simulink model "PEMFuelCellSystem"  (R2025b)
settings: Solver=VariableStepAuto  StartTime=0.0  StopTime=2500  RelTol=1e-3  AbsTol=1e-3
model workspace: external: MATLAB File PEMFuelCellSystemParameters.m (data not in the file)
values from neighbouring files (symbols this model uses):
  anode_tube_D = 0.01    [PEMFuelCellSystemParameters.m]
  cathode_tube_D = 0.05    [PEMFuelCellSystemParameters.m]
  comp_rpm_TLU = [0, 1800, 3600]    [PEMFuelCellSystemParameters.m]
  coolant_num_layers = 20    [PEMFuelCellSystemParameters.m]
  coolant_num_passes = 12    [PEMFuelCellSystemParameters.m]
  coolant_tube_D = 0.05    [PEMFuelCellSystemParameters.m]
  coolant_w_channels = 1    [PEMFuelCellSystemParameters.m]
  env_p = 0.101325    [PEMFuelCellSystemParameters.m]
  env_T = 20    [PEMFuelCellSystemParameters.m]
  N2_T = [-56.55, -50:10:-10, -5:1:5, 10:10:350]    [PEMFuelCellSystemParameters.m]
  radiator_air_area_fins = 2 * radiator_N_fins * radiator_W * radiator_gap_H    (= 11.5625)    [PEMFuelCellSystemParameters.m]
  radiator_air_area_primary = 2 * (radiator_N_tubes - 1) * radiator_W * (radiator_L + radiator_gap_H)    (= 1.223125)    [PEMFuelCellSystemParameters.m]
  radiator_eta_fin = 0.7    [PEMFuelCellSystemParameters.m]
  radiator_N_tubes = 25    [PEMFuelCellSystemParameters.m]
  radiator_rho = 2700    [PEMFuelCellSystemParameters.m]
  radiator_t_wall = 1e-4    (= 0.0001)    [PEMFuelCellSystemParameters.m]
  radiator_tube_H = 0.0015    [PEMFuelCellSystemParameters.m]
  radiator_W = 0.025    [PEMFuelCellSystemParameters.m]
  stack_area = 280    [PEMFuelCellSystemParameters.m]
  stack_iL = 1.4    [PEMFuelCellSystemParameters.m]
  stack_mea_rho = 1800    [PEMFuelCellSystemParameters.m]
  stack_num_cells = 400    [PEMFuelCellSystemParameters.m]
  stack_num_channels = 8    [PEMFuelCellSystemParameters.m]
  stack_t_gdl = 250    [PEMFuelCellSystemParameters.m]
  stack_t_membrane = 125    [PEMFuelCellSystemParameters.m]
  stack_w_channels = 1    [PEMFuelCellSystemParameters.m]
libraries: fl_lib x83, nesl_utility x23, slpidlib x2, simulink x1
(part 1 of 3)
CloseFcn:
  | try,close(h1_PEMFuelCellSystem),end
  | clear h1_PEMFuelCellSystem
  | try,close(h2_PEMFuelCellSystem),end
  | clear h2_PEMFuelCellSystem
  | try,close(h3_PEMFuelCellSystem),end
  | clear h3_PEMFuelCellSystem
  | try,close(h4_PEMFuelCellSystem),end
  | clear h4_PEMFuelCellSystem
  | try,close(h5_PEMFuelCellSystem),end
  | clear h5_PEMFuelCellSystem
  | 
  | clear tout simlog_PEMFuelCellSystem
Description:
  | PEM Fuel Cell System
settings Model: Creator=The MathWorks, Inc.  LastModifiedBy=The MathWorks, Inc.
settings SolverCC: AutoScaleAbsTol=off  MaxConsecutiveMinStep=2  AlgebraicLoopSolver=TrustRegion  MaxZcPerStep=1.0
settings DataIOCC: ReturnWorkspaceOutputs=off
settings DebuggingCC: UnconnectedInputMsg=warning  UnconnectedOutputMsg=warning  UnconnectedLineMsg=warning  SymbolicDimsDataTypeCodeGenerationDiagnostic=none
settings ModelReferenceCC: EnableRefExpFcnMdlSchedulingChecks=on
settings SFSimCC: CustomCodeUndefinedFunction=UseInterfaceOnly
settings RTWCC: GPUComputeCapability=3.5  DLArmComputeVersion=19.05
settings SimscapeCC: SimscapeLogType=all  SimscapeLogSimulationStatistics=on  SimscapeLogName=simlog_PEMFuelCellSystem  SimscapeLogDataHistory=20000.0

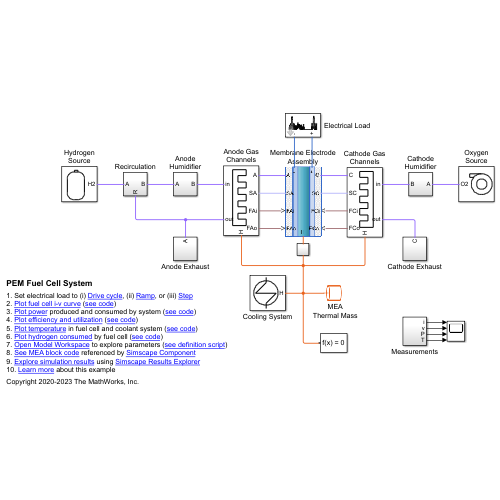
[thumbnail: Simulink's stored preview of the top-level diagram]
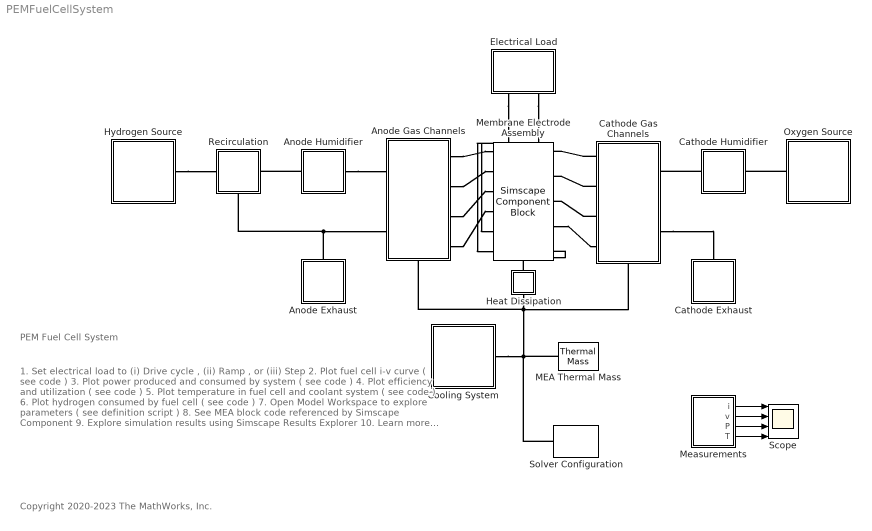
== system PEMFuelCellSystem ==
  note: PEM Fuel Cell System
  note: 1. Set electrical load to (i) Drive cycle , (ii) Ramp , or (iii) Step
      | 2. Plot fuel cell i-v curve ( see code )
      | 3. Plot power produced and consumed by system ( see code )
      | 4. Plot efficiency and utilization ( see code )
      | 5. Plot temperature in fuel cell and coolant system ( see code )
      | 6. Plot hydrogen consumed by fuel cell ( see code )
      | 7. Open Model Workspace to explore parameters ( see definition script )
      | 8. See MEA block code referenced by Simscape Component
      | 9. Explore simulation results using Simscape Results Explorer
      | 10. Learn more about this example
  note: Copyright 2020-2023 The MathWorks, Inc.
  Anode Humidifier : Subsystem  Tag=PublishSubsystem
  Anode Exhaust : Subsystem  Tag=PublishSubsystem
      settings: PortSchema="{\"entries\":[{\"content\":{\"sides\":[{\"content\":{\"connectorIds\":[]},\"type\":\"ConnectorPlacement.EquallySpacedRectSide\",\"uuid\":\"6344d1cf-22ea-4a51-9588-07afca0fac15\"},{\"content\":{\"connectorIds\":[],\"side\":\"RIGHT\"},\"type\":\"ConnectorPlacement.EquallySpacedRectSide\",\"uuid\":\"a3908f81-9410-4056-87cd-9faba76d3fb8\"},{\"content\":{\"connectorIds\":[\"LConn1\"],\"side\":\"TOP\"},\"type\":\"ConnectorPlacement.EquallySpacedRectSide\",\"uuid\":\"a1c9e24d-adb9-4361-8e9b-feafccbbdb81\"}]},\"type\":\"ConnectorPlacement.EquallySpacedConnector\",\"uuid\":\"d5180d8f-18a0-491d-9fff-909db43c9aea\"}],\"packageUris\":[\"http://schema.mathworks.com/mf0/Connector/R2020b\"],\"version\":\"1.0\"}"
  Anode Gas Channels : Subsystem  Tag=PublishSubsystem
      settings: PortSchema="{\"entries\":[{\"content\":{\"sides\":[{\"content\":{\"connectorIds\":[\"LConn1\",\"LConn2\"]},\"type\":\"ConnectorPlacement.EquallySpacedRectSide\",\"uuid\":\"f0c92738-2de1-40ac-9e4a-670524600aa2\"},{\"content\":{\"connectorIds\":[\"RConn1\",\"RConn2\",\"RConn3\",\"RConn4\"],\"side\":\"RIGHT\"},\"type\":\"ConnectorPlacement.EquallySpacedRectSide\",\"uuid\":\"f0ed995d-2dce-4bd6-9faa-b1cb502a30b1\"},{\"content\":{\"connectorIds\":[],\"side\":\"TOP\"},\"type\":\"ConnectorPlacement.EquallySpacedRectSide\",\"uuid\":\"b5d2d698-46b6-42b5-a767-bb9f1790aa28\"},{\"content\":{\"connectorIds\":[\"RConn5\"],\"side\":\"BOTTOM\"},\"type\":\"ConnectorPlacement.EquallySpacedRectSide\",\"uuid\":\"3e8c99a3-0044-43a9-bacb-b652445e4ac6\"}]},\"type\":\"ConnectorPlacement.EquallySpacedConnector\",\"uuid\":\"912925fb-ca80-4fe6-8a1d-a2308cfd6f88\"}],\"packageUris\":[\"http://schema.mathworks.com/mf0/Connector/R2020b\"],\"version\":\"1.0\"}"
      mask Display:
      | plot(0, 0)
      | plot(100, 100)
      | 
      | x1 = 25;
      | x2 = 65;
      | y1 = 23;
      | y2 = 95;
      | xt = 15;
      | yt = 9;
      | 
      | x_pattern = [x2 x2    x1+xt x1+xt   x1+xt   x2     ];
      | y_pattern = [y2 y2-yt y2-yt y2-2*yt y2-2*yt y2-2*yt];
      | 
      | plot([x1 x1 x2 x_pattern x_pattern      x_pattern      x_pattern         x2    x1], ...
      |      [y1-yt y2 y2 y_pattern y_pattern-2*yt y_pattern-4*yt y_pattern-6*yt y1-yt y1-yt])
  Cathode Humidifier : Subsystem  Tag=PublishSubsystem
  Cathode Exhaust : Subsystem  Tag=PublishSubsystem
      settings: PortSchema="{\"entries\":[{\"content\":{\"sides\":[{\"content\":{\"connectorIds\":[]},\"type\":\"ConnectorPlacement.EquallySpacedRectSide\",\"uuid\":\"6344d1cf-22ea-4a51-9588-07afca0fac15\"},{\"content\":{\"connectorIds\":[],\"side\":\"RIGHT\"},\"type\":\"ConnectorPlacement.EquallySpacedRectSide\",\"uuid\":\"a3908f81-9410-4056-87cd-9faba76d3fb8\"},{\"content\":{\"connectorIds\":[\"LConn1\"],\"side\":\"TOP\"},\"type\":\"ConnectorPlacement.EquallySpacedRectSide\",\"uuid\":\"a1c9e24d-adb9-4361-8e9b-feafccbbdb81\"}]},\"type\":\"ConnectorPlacement.EquallySpacedConnector\",\"uuid\":\"d5180d8f-18a0-491d-9fff-909db43c9aea\"}],\"packageUris\":[\"http://schema.mathworks.com/mf0/Connector/R2020b\"],\"version\":\"1.0\"}"
  Cathode Gas Channels : Subsystem  Tag=PublishSubsystem
      settings: PortSchema="{\"entries\":[{\"content\":{\"sides\":[{\"content\":{\"connectorIds\":[\"LConn1\",\"LConn2\",\"LConn3\",\"LConn4\"]},\"type\":\"ConnectorPlacement.EquallySpacedRectSide\",\"uuid\":\"d09155df-6760-40de-80f3-d532399b6b43\"},{\"content\":{\"connectorIds\":[\"RConn1\",\"RConn2\"],\"side\":\"RIGHT\"},\"type\":\"ConnectorPlacement.EquallySpacedRectSide\",\"uuid\":\"8f76bd4e-30c2-4c8b-860a-78c10353bd22\"},{\"content\":{\"connectorIds\":[],\"side\":\"TOP\"},\"type\":\"ConnectorPlacement.EquallySpacedRectSide\",\"uuid\":\"7de91a32-4f26-479e-bbec-b6009a288b8f\"},{\"content\":{\"connectorIds\":[\"RConn3\"],\"side\":\"BOTTOM\"},\"type\":\"ConnectorPlacement.EquallySpacedRectSide\",\"uuid\":\"b696b46e-4734-4c8a-bae1-7c8793078c6b\"}]},\"type\":\"ConnectorPlacement.EquallySpacedConnector\",\"uuid\":\"30d7c265-b676-4649-8112-8a94c6c095da\"}],\"packageUris\":[\"http://schema.mathworks.com/mf0/Connector/R2020b\"],\"version\":\"1.0\"}"
      mask Display:
      | plot(0, 0)
      | plot(100, 100)
      | 
      | x1 = 35;
      | x2 = 75;
      | y1 = 23;
      | y2 = 95;
      | xt = 15;
      | yt = 9;
      | 
      | x_pattern = [x1 x1    x2-xt x2-xt   x2-xt   x1     ];
      | y_pattern = [y2 y2-yt y2-yt y2-2*yt y2-2*yt y2-2*yt];
      | 
      | plot([x2 x2 x1 x_pattern x_pattern      x_pattern      x_pattern         x1    x2], ...
      |      [y1-yt y2 y2 y_pattern y_pattern-2*yt y_pattern-4*yt y_pattern-6*yt y1-yt y1-yt])
  Cooling System : Subsystem  Tag=PublishSubsystem
      mask Display:
      | plot(0, 0)
      | plot(100, 100)
      | 
      | n = 80;
      | r = 35;
      | 
      | x = 45;
      | y = 50;
      | t = 5;
      | 
      | plot(cos(linspace(0, 2*pi, n))*r + x, sin(linspace(0, 2*pi, n))*r + y)
      | 
      | plot([x x x-r+t x+r-t x x], [y+r+2*t y+r-t y y y-r+t y-r-2*t])
  Electrical Load : Subsystem  Tag=PublishSubsystem  mask(Electrical Load){input_type=Drive cycle}
      mask prompts: input_type "Select one of the following scenarios:"
      settings: PortSchema="{\"entries\":[{\"content\":{\"sides\":[{\"content\":{\"connectorIds\":[]},\"type\":\"ConnectorPlacement.EquallySpacedRectSide\",\"uuid\":\"cf26c57a-4aaa-4eca-a1cf-dab3379228b7\"},{\"content\":{\"connectorIds\":[],\"side\":\"RIGHT\"},\"type\":\"ConnectorPlacement.EquallySpacedRectSide\",\"uuid\":\"bd4a28c6-f8d3-4492-9f61-a12eb17ccdd3\"},{\"content\":{\"connectorIds\":[],\"side\":\"TOP\"},\"type\":\"ConnectorPlacement.EquallySpacedRectSide\",\"uuid\":\"7f54a4db-ccf4-4e3a-a135-4ada067d241f\"},{\"content\":{\"connectorIds\":[\"RConn1\",\"RConn2\"],\"side\":\"BOTTOM\"},\"type\":\"ConnectorPlacement.EquallySpacedRectSide\",\"uuid\":\"8817983d-3f79-43b3-9594-6d12f7dcf066\"}]},\"type\":\"ConnectorPlacement.EquallySpacedConnector\",\"uuid\":\"79253ea6-cd7f-4983-840a-f5cee3a4dd91\"}],\"packageUris\":[\"http://schema.mathworks.com/mf0/Connector/R2020b\"],\"version\":\"1.0\"}"
      mask TypeOptions input_type: Drive cycle | Ramp | Step
      mask Callback input_type:
      | activeVariant = get_param(gcb, 'input_type');
      | set_param([gcb '/Inputs'], 'OverrideUsingVariant', activeVariant)
      mask Display:
      | blk = get_param([gcb, '/Inputs'], 'CompiledActiveChoiceBlock');
      | eval(get_param(blk, 'MaskDisplay'))
  Heat Dissipation : Subsystem
      settings: PortSchema="{\"entries\":[{\"content\":{\"sides\":[{\"content\":{\"connectorIds\":[]},\"type\":\"ConnectorPlacement.EquallySpacedRectSide\",\"uuid\":\"40b2385a-b20e-464f-8016-3228e4acac4a\"},{\"content\":{\"connectorIds\":[],\"side\":\"RIGHT\"},\"type\":\"ConnectorPlacement.EquallySpacedRectSide\",\"uuid\":\"0e95dc4b-d2da-4ab6-a6e9-e2cb275776ce\"},{\"content\":{\"connectorIds\":[\"LConn1\"],\"side\":\"TOP\"},\"type\":\"ConnectorPlacement.EquallySpacedRectSide\",\"uuid\":\"0f5995c7-26f6-433d-889b-dea78bcd2b2a\"},{\"content\":{\"connectorIds\":[\"RConn1\"],\"side\":\"BOTTOM\"},\"type\":\"ConnectorPlacement.EquallySpacedRectSide\",\"uuid\":\"a2ee1c19-f9e9-4dbd-a9ff-92feea387e85\"}]},\"type\":\"ConnectorPlacement.EquallySpacedConnector\",\"uuid\":\"721753ea-9ada-4c74-8c6f-50b905d96904\"}],\"packageUris\":[\"http://schema.mathworks.com/mf0/Connector/R2020b\"],\"version\":\"1.0\"}"
  Hydrogen Source : Subsystem  Tag=PublishSubsystem
      mask Display:
      | plot(0, 0)
      | plot(100, 100)
      | 
      | n = 20;
      | r = 20;
      | x1 = 15;
      | x2 = 65;
      | y1 = 5;
      | y2 = 85;
      | 
      | plot([x1 x1], [y1+r y2-r])
      | plot([x1+r x2-r], [y2 y2])
      | plot([x2 x2], [y2-r y1+r])
      | plot([x2-r x1+r], [y1 y1])
      | 
      | plot(cos(linspace(pi/2, pi, n))*r + x1+r, sin(linspace(pi/2, pi, n))*r + y2-r)
      | plot(cos(linspace(0, pi/2, n))*r + x2-r, sin(linspace(0, pi/2, n))*r + y2-r)
      | plot(cos(linspace(3*pi/2, 2*pi, n))*r + x2-r, sin(linspace(3*pi/2, 2*pi, n))*r + y1+r)
      | plot(cos(linspace(pi, 3*pi/2, n))*r + x1+r, sin(linspace(pi, 3*pi/2, n))*r + y1+r)
      | 
      | plot([-5 -5 5 5] + (x1+x2)/2, [0 5 5 0] + y2)
  MEA Thermal Mass : fl_lib/Thermal/Thermal Elements/Thermal Mass  mass_type=foundation.enum.constant_variable.constant  mass=stack_mea_rho * stack_area*1e-4 * (stack_t_membrane + 2*stack_t_gdl)*1e-6 * stack_num_cells kg  sp_heat=stack_mea_cp J/kg/K  mass_min=1e-6 kg  num_ports=foundation.enum.numPorts2.one  m_specify=off  m_priority=High  m=1 kg  m_nominal_specify=off  m_nominal_value=1  m_nominal_unit=kg  T_specify=on  T_priority=High  T=env_T degC  T_nominal_specify=off  T_nominal_value=1  T_nominal_unit=K  Q_specify=off  Q_priority=None  Q=0 W  Q_nominal_specify=off  Q_nominal_value=1  Q_nominal_unit=W
  Measurements : Subsystem
  Membrane Electrode Assembly : SimscapeComponentBlock  SourceFile=FuelCell  ComponentPath=FuelCell  ComponentVariants="[\"FuelCell\"]"  ComponentVariantNames="[\"FuelCell\"]"  ClassName=FuelCell  SchemaVersion=1  N_cell=stack_num_cells  area_cell=stack_area cm^2  t_membrane=stack_t_membrane um  t_gdl_A=stack_t_gdl um  t_gdl_C=stack_t_gdl um  io=stack_io A/cm^2  iL=stack_iL A/cm^2  alpha=stack_alpha  D_H2O_gdl_A=stack_D_gdl cm^2/s  D_H2O_gdl_C=stack_D_gdl cm^2/s  rho_membrane=stack_membrane_rho kg/m^3  M_membrane=stack_membrane_MW kg/mol  i_specify=off  i_priority=None  i=0 A  i_nominal_specify=off  i_nominal_value=1  i_nominal_unit=A  Q_specify=off  Q_priority=None  Q=0 W  Q_nominal_specify=off  Q_nominal_value=1  Q_nominal_unit=W  a_H2O_acl_specify=off  a_H2O_acl_priority=None  a_H2O_acl=0.5  a_H2O_acl_nominal_specify=off  a_H2O_acl_nominal_value=1  a_H2O_acl_nominal_unit=1  a_H2O_ccl_specify=off  a_H2O_ccl_priority=None  a_H2O_ccl=0.5  a_H2O_ccl_nominal_specify=off  a_H2O_ccl_nominal_value=1  a_H2O_ccl_nominal_unit=1
      settings: CopyFcn=simscape.sscblock.internal.componentBlockCallback(gcbh,'COPY')  PreCopyFcn=simscape.sscblock.internal.componentBlockCallback(gcbh,'PRECOPY')  PreDeleteFcn=simscape.sscblock.internal.componentBlockCallback(gcbh,'PREDELETE')  InternalSimscapePortConfiguration="{\"Bottom\":[{\"id\":\"H\",\"label\":\"H\",\"type\":\"foundation.thermal.thermal\"}],\"Left\":[{\"id\":\"A\",\"label\":\"A\",\"type\":\"foundation.moist_air.moist_air\"},{\"id\":\"SA\",\"label\":\"SA\",\"type\":\"foundation.moist_air.moist_air_source\"},{\"id\":\"FAi\",\"label\":\"FAi\",\"type\":\"input\"},{\"id\":\"FAo\",\"label\":\"FAo\",\"type\":\"input\"}],\"Right\":[{\"id\":\"C\",\"label\":\"C\",\"type\":\"foundation.moist_air.moist_air\"},{\"id\":\"SC\",\"label\":\"SC\",\"type\":\"foundation.moist_air.moist_air_source\"},{\"id\":\"FCi\",\"label\":\"FCi\",\"type\":\"input\"},{\"id\":\"FCo\",\"label\":\"FCo\",\"type\":\"input\"}],\"Top\":[{\"id\":\"n\",\"label\":\"-\",\"type\":\"foundation.electrical.electrical\"},{\"id\":\"p\",\"label\":\"+\",\"type\":\"foundation.electrical.electrical\"}]}"
      mask Type: Fuel Cell
  Oxygen Source : Subsystem  Tag=PublishSubsystem
      mask Display:
      | plot(0, 0)
      | plot(100, 100)
      | 
      | n = 80;
      | r1 = 15;
      | r2 = 30;
      | 
      | plot(cos(linspace(0, 2*pi, n))*r1 + 65, sin(linspace(0, 2*pi, n))*r1 + 50)
      | plot(cos(linspace(0, 2*pi, n))*r2 + 65, sin(linspace(0, 2*pi, n))*r2 + 50)
      | 
      | plot([65 30 30 42], [80 80 70 70])
  Recirculation : Subsystem  Tag=PublishSubsystem
      settings: PortSchema="{\"entries\":[{\"content\":{\"sides\":[{\"content\":{\"connectorIds\":[\"LConn1\"]},\"type\":\"ConnectorPlacement.EquallySpacedRectSide\",\"uuid\":\"a905d28b-4136-4e4b-b56f-ff4ef454860e\"},{\"content\":{\"connectorIds\":[\"RConn1\"],\"side\":\"RIGHT\"},\"type\":\"ConnectorPlacement.EquallySpacedRectSide\",\"uuid\":\"7d453241-460d-4f71-8108-f868ae96b726\"},{\"content\":{\"connectorIds\":[],\"side\":\"TOP\"},\"type\":\"ConnectorPlacement.EquallySpacedRectSide\",\"uuid\":\"5de5a8e7-eaa9-43ea-9e3e-e109b24be5c4\"},{\"content\":{\"connectorIds\":[\"RConn2\"],\"side\":\"BOTTOM\"},\"type\":\"ConnectorPlacement.EquallySpacedRectSide\",\"uuid\":\"9c44ad98-d3d2-40d8-a226-ad16e20687d9\"}]},\"type\":\"ConnectorPlacement.EquallySpacedConnector\",\"uuid\":\"be431bc9-ad83-41b5-a4a3-7fe11e97fedb\"}],\"packageUris\":[\"http://schema.mathworks.com/mf0/Connector/R2020b\"],\"version\":\"1.0\"}"
  Scope : Scope  NumInputPorts=4
      settings: Title=Current (A)  ActiveDisplayYMinimum=-34.06707  ActiveDisplayYMaximum=306.60365
  Solver Configuration : nesl_utility/Solver Configuration  PhysicalDomain=network_engine_domain  SubClassName=solver  LeftPortType=input  RightPortType=generic  Tones=[]  Harmonics=[]  SimulateNoise=off  Profile=off  UseLocalSampling=off  EnableSwitchedLinearOptims=on  FrequencyDomain=off  UseCCode=off  RelTol=0.001  AbsTol=1e-06  MinStep=1e-09  ToWorkspace=off  RevertToSquareIcSolve=off  NumHomotopyIterations=100  PhasorMode=off  PhasorModeNumHarmonics=1  ConsistencySolver=NEWTON_XTOL_AFTER_FTOL  IndexReductionMethod=DerivativeReplacement  DoDC=off  ResidualTolerance=1e-09  ConsistencyTolSource=GLOBAL  ConsistencyAbsTol=0.001  ConsistencyRelTol=0.001  ConsistencyTolFactor=0.001  UseLocalSolver=off  LocalSolverChoice=NE_BACKWARD_EULER_ADVANCER  ResolveIndetEquations=on  FunctionEvalNumThread=1  LocalSolverSampleTime=0.001  DoFixedCost=off  MaxNonlinIter=3  MaxModeIter=2  ComputeImpulses=off  ImpulseIterations=2  LinearAlgebra=auto  LinearAlgebraNumThread=0  EquationFormulation=NE_TIME_EF  DelaysMemoryBudget=1024  AutomaticFiltering=on  FilteringTimeConstant=0.001  PartitionStorageMethod=AS_NEEDED  PartitionMemoryBudget=1024  PartitionMethod=ROBUST  MultibodyUseLocalSolver=off  MultibodyLocalSolverChoice=ODE1  MultibodyLocalSolverSampleTime=0.001
  wires:
  Measurements/1(i) -> Scope/1
  Measurements/2(v) -> Scope/2
  Measurements/3(P) -> Scope/3
  Measurements/4(T) -> Scope/4
  connections:
  Cathode Gas Channels/RConn2 -- Cathode Exhaust/LConn1
  Cathode Humidifier/LConn1 -- Cathode Gas Channels/RConn1
  Anode Gas Channels/RConn1 -- Membrane Electrode Assembly/LConn1
  Anode Gas Channels/RConn2 -- Membrane Electrode Assembly/LConn2
  Anode Gas Channels/RConn3 -- Membrane Electrode Assembly/LConn3
  Cathode Gas Channels/LConn1 -- Membrane Electrode Assembly/RConn1
  Cathode Gas Channels/LConn2 -- Membrane Electrode Assembly/RConn2
  Cathode Gas Channels/LConn3 -- Membrane Electrode Assembly/RConn3
  Anode Exhaust/LConn1 -- Recirculation/RConn2 -- Anode Gas Channels/LConn2
  Oxygen Source/LConn1 -- Cathode Humidifier/RConn1
  Electrical Load/RConn1 -- Membrane Electrode Assembly/LConn5
  Electrical Load/RConn2 -- Membrane Electrode Assembly/LConn6
  Anode Gas Channels/RConn4 -- Membrane Electrode Assembly/LConn4
  Membrane Electrode Assembly/RConn4 -- Cathode Gas Channels/LConn4
  Anode Humidifier/RConn1 -- Anode Gas Channels/LConn1
  Hydrogen Source/RConn1 -- Recirculation/LConn1
  Anode Humidifier/LConn1 -- Recirculation/RConn1
  MEA Thermal Mass/LConn1 -- Solver Configuration/RConn1 -- Heat Dissipation/RConn1 -- Anode Gas Channels/RConn5 -- Cathode Gas Channels/RConn3 -- Cooling System/RConn1
  Heat Dissipation/LConn1 -- Membrane Electrode Assembly/RConn5

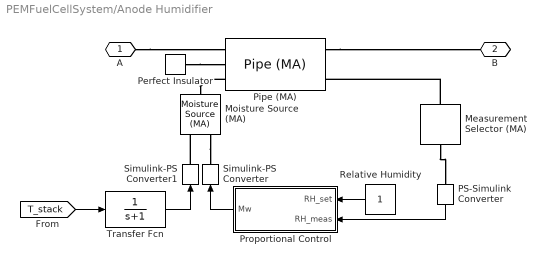
== system PEMFuelCellSystem/Anode Humidifier ==
  Measurement Selector (MA) : fl_lib/Moist Air/Sensors/Measurement Selector (MA)  moisture_spec=foundation.enum.moisture_spec.relative_humidity  trace_gas_spec=foundation.enum.trace_gas_spec.mole_fraction
      settings: InternalSimscapePortConfiguration="{\"Bottom\":[],\"Left\":[{\"id\":\"F\",\"label\":\"F\",\"type\":\"input\"}],\"Right\":[{\"id\":\"P\",\"label\":\"P\",\"type\":\"output\"},{\"id\":\"T\",\"label\":\"T\",\"type\":\"output\"},{\"id\":\"W\",\"label\":\"W\",\"type\":\"output\"},{\"id\":\"G\",\"label\":\"G\",\"type\":\"output\"},{\"id\":\"D\",\"label\":\"D\",\"type\":\"output\"}],\"Top\":[]}"
  Moisture Source (MA) : fl_lib/Moist Air/Sources/Moisture & Trace Gas Sources/Moisture Source (MA)  source_type=foundation.enum.constant_controlled.controlled  moisture_source_spec=foundation.enum.MoistureSourceSpec.WaterVapor  vapor_from_liquid=false  moisture_mass_flow=0 kg/s  temperature_spec=foundation.enum.temperature_spec.atmospheric  moisture_temperature=293.15 K  Phi_S_specify=off  Phi_S_priority=None  Phi_S=0 kW  Phi_S_nominal_specify=off  Phi_S_nominal_value=1  Phi_S_nominal_unit=kW  mdot_w_S_specify=off  mdot_w_S_priority=None  mdot_w_S=0 kg/s  mdot_w_S_nominal_specify=off  mdot_w_S_nominal_value=1  mdot_w_S_nominal_unit=kg/s  mdot_d_S_specify=off  mdot_d_S_priority=None  mdot_d_S=0 kg/s  mdot_d_S_nominal_specify=off  mdot_d_S_nominal_value=1  mdot_d_S_nominal_unit=kg/s
      settings: InternalSimscapePortConfiguration="{\"Bottom\":[],\"Left\":[{\"id\":\"S\",\"label\":\"S\",\"type\":\"foundation.moist_air.moist_air_source\"}],\"Right\":[{\"id\":\"M\",\"label\":\"M\",\"type\":\"input\"},{\"id\":\"T\",\"label\":\"T\",\"type\":\"input\"}],\"Top\":[]}"
  PS-Simulink Converter : nesl_utility/PS-Simulink Converter  PhysicalDomain=network_engine_domain  SubClassName=ps_output  LeftPortType=input  RightPortType=output  PseudoPeriodic=off  Frequencies=[]  VectorFormat=1-D array  Unit=1  AffineConversion=off
  Perfect Insulator : fl_lib/Thermal/Thermal Elements/Perfect Insulator  T_specify=off  T_priority=None  T=0 K  T_nominal_specify=off  T_nominal_value=1  T_nominal_unit=K
  Pipe (MA) : fl_lib/Moist Air/Elements/Pipe (MA)  length=0.25 m  area=pi*0.05^2/4 m^2  Dh=0.05 m  length_add=0.1 m  roughness=15e-6 m  Re_lam=2000  Re_tur=4000  shape_factor=64  Nu_lam=3.66  wall_condensation=simscape.enum.onoff.off  RH_ws=1  time_constant_cond=1e-3 s  time_constant_evap=1e-3 s  fraction_entrained=1  moisture_trace_gas_source=foundation.enum.moisture_trace_gas_source.controlled  moisture_source_spec=foundation.enum.MoistureSourceSpec.WaterVapor  vapor_from_liquid=false  moisture_mass_flow=0 kg/s  moisture_temperature_spec=foundation.enum.temperature_spec.atmospheric  moisture_temperature=293.15 K  trace_gas_mass_flow=0 kg/s  trace_gas_temperature_spec=foundation.enum.temperature_spec.atmospheric  trace_gas_temperature=293.15 K  p_init=env_p MPa  p_init_priority=foundation.enum.Priority.High  T_init=env_T degC  T_init_priority=foundation.enum.Priority.High  humidity_spec=foundation.enum.HumiditySpec.RelativeHumidity  RH_init=0  RH_init_priority=foundation.enum.Priority.High  x_w_init=0  x_w_init_priority=foundation.enum.Priority.None  y_w_init=0  y_w_init_priority=foundation.enum.Priority.None  HR_init=0  HR_init_priority=foundation.enum.Priority.None  Tw_init=287 K  Tw_init_priority=foundation.enum.Priority.High  trace_gas_spec=foundation.enum.trace_gas_spec.mole_fraction  x_g_init=0  x_g_init_priority=foundation.enum.Priority.None  y_g_init=tank_yH2  y_g_init_priority=foundation.enum.Priority.High  r_d_init=0  r_d_init_priority=foundation.enum.Priority.High
      settings: InternalSimscapePortConfiguration="{\"Bottom\":[],\"Left\":[{\"id\":\"A\",\"label\":\"A\",\"type\":\"foundation.moist_air.moist_air\"},{\"id\":\"H\",\"label\":\"H\",\"type\":\"foundation.thermal.thermal\"},{\"id\":\"S\",\"label\":\"S\",\"type\":\"foundation.moist_air.moist_air_source\"}],\"Right\":[{\"id\":\"B\",\"label\":\"B\",\"type\":\"foundation.moist_air.moist_air\"},{\"id\":\"W\",\"label\":\"W\",\"type\":\"output\"},{\"id\":\"F\",\"label\":\"F\",\"type\":\"output\"}],\"Top\":[]}"
  Proportional Control : Subsystem
  Relative Humidity : Constant
  Simulink-PS Converter : nesl_utility/Simulink-PS Converter  PhysicalDomain=network_engine_domain  SubClassName=ps_input  LeftPortType=input  RightPortType=output  PseudoPeriodic=off  Frequencies=[]  NoiseDistribution=none  NoiseParameters=[]  Unit=kg/s  AffineConversion=off  FilteringAndDerivatives=provide  SimscapeFilterOrder=1  InputFilterTimeConstant=0.001  UdotUserProvided=0
  Simulink-PS Converter1 : nesl_utility/Simulink-PS Converter  PhysicalDomain=network_engine_domain  SubClassName=ps_input  LeftPortType=input  RightPortType=output  PseudoPeriodic=off  Frequencies=[]  NoiseDistribution=none  NoiseParameters=[]  Unit=degC  AffineConversion=on  FilteringAndDerivatives=provide  SimscapeFilterOrder=1  InputFilterTimeConstant=0.001  UdotUserProvided=0
  Transfer Fcn : TransferFcn  Denominator=[1 1]
  A : PMIOPort  Side=Left
  B : PMIOPort  Port=2  Side=Right
  wires:
  Transfer Fcn/1 -> Simulink-PS Converter1/1
  [T_stack] -> Transfer Fcn/1
  Relative Humidity/1 -> Proportional Control/1(RH_set)
  PS-Simulink Converter/1 -> Proportional Control/2(RH_meas)
  Proportional Control/1(Mw) -> Simulink-PS Converter/1
  connections:
  Moisture Source (MA)/RConn1 -- Simulink-PS Converter/RConn1
  Measurement Selector (MA)/LConn1 -- Pipe (MA)/RConn3
  Simulink-PS Converter1/RConn1 -- Moisture Source (MA)/RConn2
  Pipe (MA)/LConn3 -- Moisture Source (MA)/LConn1
  Perfect Insulator/LConn1 -- Pipe (MA)/LConn2
  Pipe (MA)/RConn1 -- B/RConn1
  A/RConn1 -- Pipe (MA)/LConn1
  Measurement Selector (MA)/RConn3 -- PS-Simulink Converter/LConn1

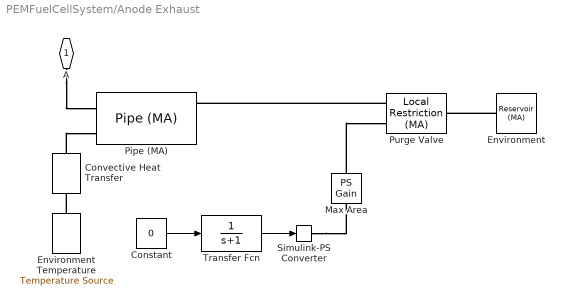
== system PEMFuelCellSystem/Anode Exhaust ==
  Constant : Constant  Value=0
  Convective Heat Transfer : fl_lib/Thermal/Thermal Elements/Convective Heat Transfer  thermal_type=foundation.enum.constant_variable.constant  area=pi*anode_tube_D*1 m^2  heat_tr_coeff=20 W/(m^2 * K)  min_heat_tr_coeff=1e-3 W/(K*m^2)  T_specify=off  T_priority=None  T=0 K  T_nominal_specify=off  T_nominal_value=1  T_nominal_unit=K  Q_specify=off  Q_priority=None  Q=0 W  Q_nominal_specify=off  Q_nominal_value=1  Q_nominal_unit=W
  Environment : fl_lib/Moist Air/Elements/Reservoir (MA)  pressure_input=false  pressure_spec=foundation.enum.pressure_spec.specified  reservoir_pressure=env_p MPa  temperature_input=false  temperature_spec=foundation.enum.temperature_spec.specified  reservoir_temperature=env_T degC  humidity_input=false  humidity_spec=foundation.enum.HumiditySpec.RelativeHumidity  reservoir_RH=0  reservoir_x_w=0.01  reservoir_y_w=0.01  reservoir_HR=0.01  reservoir_Tw=287 K  trace_gas_input=false  trace_gas_spec=foundation.enum.trace_gas_spec.mole_fraction  reservoir_x_g=0.001  reservoir_y_g=tank_yH2  water_droplets_input=false  reservoir_r_d=0  RH_ws=1  area_A=pi*anode_tube_D^2/4 m^2  input_error_spec=foundation.enum.input_range_error.warn
  Environment Temperature : fl_lib/Thermal/Thermal Sources/Temperature Source  temperature=env_T degC
  Max Area : fl_lib/Physical Signals/Functions/PS Gain  gain=pi*(0.2*anode_tube_D)^2/4 m^2
  Pipe (MA) : fl_lib/Moist Air/Elements/Pipe (MA)  length=1 m  area=pi*anode_tube_D^2/4 m^2  Dh=anode_tube_D m  length_add=0.1 m  roughness=15e-6 m  Re_lam=2000  Re_tur=4000  shape_factor=64  Nu_lam=3.66  wall_condensation=simscape.enum.onoff.off  RH_ws=1  time_constant_cond=1e-3 s  time_constant_evap=1e-3 s  fraction_entrained=1  moisture_trace_gas_source=foundation.enum.moisture_trace_gas_source.none  moisture_source_spec=foundation.enum.MoistureSourceSpec.WaterVapor  vapor_from_liquid=false  moisture_mass_flow=0 kg/s  moisture_temperature_spec=foundation.enum.temperature_spec.atmospheric  moisture_temperature=293.15 K  trace_gas_mass_flow=0 kg/s  trace_gas_temperature_spec=foundation.enum.temperature_spec.atmospheric  trace_gas_temperature=293.15 K  p_init=env_p MPa  p_init_priority=foundation.enum.Priority.High  T_init=env_T degC  T_init_priority=foundation.enum.Priority.High  humidity_spec=foundation.enum.HumiditySpec.RelativeHumidity  RH_init=0  RH_init_priority=foundation.enum.Priority.High  x_w_init=0  x_w_init_priority=foundation.enum.Priority.None  y_w_init=0  y_w_init_priority=foundation.enum.Priority.None  HR_init=0  HR_init_priority=foundation.enum.Priority.None  Tw_init=287 K  Tw_init_priority=foundation.enum.Priority.High  trace_gas_spec=foundation.enum.trace_gas_spec.mole_fraction  x_g_init=0  x_g_init_priority=foundation.enum.Priority.None  y_g_init=tank_yH2  y_g_init_priority=foundation.enum.Priority.High  r_d_init=0  r_d_init_priority=foundation.enum.Priority.High
  Purge Valve : fl_lib/Moist Air/Elements/Local Restriction (MA)  restriction_type=foundation.enum.restriction_type.variable  restriction_area=0.001 m^2  min_area=pi*(1e-4*anode_tube_D)^2/4 m^2  max_area=pi*(0.2*anode_tube_D)^2/4 m^2  area=pi*anode_tube_D^2/4 m^2  Cd=0.64  B_lam=0.999
  Simulink-PS Converter : nesl_utility/Simulink-PS Converter  PhysicalDomain=network_engine_domain  SubClassName=ps_input  LeftPortType=input  RightPortType=output  PseudoPeriodic=off  Frequencies=[]  NoiseDistribution=none  NoiseParameters=[]  Unit=1  AffineConversion=off  FilteringAndDerivatives=provide  SimscapeFilterOrder=1  InputFilterTimeConstant=0.001  UdotUserProvided=0
  Transfer Fcn : TransferFcn  Denominator=[1 1]
  A : PMIOPort  Side=Left
  wires:
  Constant/1 -> Transfer Fcn/1
  Transfer Fcn/1 -> Simulink-PS Converter/1
  connections:
  Environment/LConn1 -- Purge Valve/RConn1
  A/RConn1 -- Pipe (MA)/LConn1
  Purge Valve/LConn1 -- Pipe (MA)/RConn1
  Simulink-PS Converter/RConn1 -- Max Area/LConn1
  Max Area/RConn1 -- Purge Valve/LConn2
  Convective Heat Transfer/LConn1 -- Pipe (MA)/LConn2
  Environment Temperature/LConn1 -- Convective Heat Transfer/RConn1

== system PEMFuelCellSystem/Anode Gas Channels ==
  note: connection to share anode fluid properties only
  Pipe (MA) : fl_lib/Moist Air/Elements/Pipe (MA)  length=sqrt(stack_area) / 2 cm  area=stack_w_channels^2 * stack_num_channels * stack_num_cells cm^2  Dh=stack_w_channels cm  length_add=1 cm  roughness=15e-6 m  Re_lam=2000  Re_tur=4000  shape_factor=64  Nu_lam=3.66  wall_condensation=simscape.enum.onoff.off  RH_ws=1  time_constant_cond=1e-3 s  time_constant_evap=1e-3 s  fraction_entrained=1  moisture_trace_gas_source=foundation.enum.moisture_trace_gas_source.none  moisture_source_spec=foundation.enum.MoistureSourceSpec.WaterVapor  vapor_from_liquid=false  moisture_mass_flow=0 kg/s  moisture_temperature_spec=foundation.enum.temperature_spec.atmospheric  moisture_temperature=293.15 K  trace_gas_mass_flow=0 kg/s  trace_gas_temperature_spec=foundation.enum.temperature_spec.atmospheric  trace_gas_temperature=293.15 K  p_init=env_p MPa  p_init_priority=foundation.enum.Priority.High  T_init=env_T degC  T_init_priority=foundation.enum.Priority.High  humidity_spec=foundation.enum.HumiditySpec.RelativeHumidity  RH_init=0  RH_init_priority=foundation.enum.Priority.High  x_w_init=0  x_w_init_priority=foundation.enum.Priority.None  y_w_init=0  y_w_init_priority=foundation.enum.Priority.None  HR_init=0  HR_init_priority=foundation.enum.Priority.None  Tw_init=287 K  Tw_init_priority=foundation.enum.Priority.High  trace_gas_spec=foundation.enum.trace_gas_spec.mole_fraction  x_g_init=0  x_g_init_priority=foundation.enum.Priority.None  y_g_init=tank_yH2  y_g_init_priority=foundation.enum.Priority.High  r_d_init=0  r_d_init_priority=foundation.enum.Priority.High
  Pipe (MA)1 : fl_lib/Moist Air/Elements/Pipe (MA)  length=sqrt(stack_area) / 2 cm  area=stack_w_channels^2 * stack_num_channels * stack_num_cells cm^2  Dh=stack_w_channels cm  length_add=1 cm  roughness=15e-6 m  Re_lam=2000  Re_tur=4000  shape_factor=64  Nu_lam=3.66  wall_condensation=simscape.enum.onoff.off  RH_ws=1  time_constant_cond=1e-3 s  time_constant_evap=1e-3 s  fraction_entrained=1  moisture_trace_gas_source=foundation.enum.moisture_trace_gas_source.controlled  moisture_source_spec=foundation.enum.MoistureSourceSpec.WaterVapor  vapor_from_liquid=false  moisture_mass_flow=0 kg/s  moisture_temperature_spec=foundation.enum.temperature_spec.atmospheric  moisture_temperature=293.15 K  trace_gas_mass_flow=0 kg/s  trace_gas_temperature_spec=foundation.enum.temperature_spec.atmospheric  trace_gas_temperature=293.15 K  p_init=env_p MPa  p_init_priority=foundation.enum.Priority.High  T_init=env_T degC  T_init_priority=foundation.enum.Priority.High  humidity_spec=foundation.enum.HumiditySpec.RelativeHumidity  RH_init=0  RH_init_priority=foundation.enum.Priority.High  x_w_init=0  x_w_init_priority=foundation.enum.Priority.None  y_w_init=0  y_w_init_priority=foundation.enum.Priority.None  HR_init=0  HR_init_priority=foundation.enum.Priority.None  Tw_init=287 K  Tw_init_priority=foundation.enum.Priority.High  trace_gas_spec=foundation.enum.trace_gas_spec.mole_fraction  x_g_init=0  x_g_init_priority=foundation.enum.Priority.None  y_g_init=tank_yH2  y_g_init_priority=foundation.enum.Priority.High  r_d_init=0  r_d_init_priority=foundation.enum.Priority.High
      settings: InternalSimscapePortConfiguration="{\"Bottom\":[],\"Left\":[{\"id\":\"A\",\"label\":\"A\",\"type\":\"foundation.moist_air.moist_air\"},{\"id\":\"H\",\"label\":\"H\",\"type\":\"foundation.thermal.thermal\"},{\"id\":\"S\",\"label\":\"S\",\"type\":\"foundation.moist_air.moist_air_source\"}],\"Right\":[{\"id\":\"B\",\"label\":\"B\",\"type\":\"foundation.moist_air.moist_air\"},{\"id\":\"W\",\"label\":\"W\",\"type\":\"output\"},{\"id\":\"F\",\"label\":\"F\",\"type\":\"output\"}],\"Top\":[]}"
  in : PMIOPort  Side=Left
  out : PMIOPort  Port=2  Side=Left
  A : PMIOPort  Port=3  Side=Right
  SA : PMIOPort  Port=4  Side=Right
  FAi : PMIOPort  Port=5  Side=Right
  FAo : PMIOPort  Port=6  Side=Right
  H : PMIOPort  Port=7  Side=Right
  connections:
  Pipe (MA)/LConn1 -- in/RConn1
  Pipe (MA)1/RConn1 -- out/RConn1
  Pipe (MA)/LConn2 -- Pipe (MA)1/LConn2 -- H/RConn1
  FAo/RConn1 -- Pipe (MA)1/RConn3
  Pipe (MA)/RConn3 -- FAi/RConn1
  Pipe (MA)1/LConn3 -- SA/RConn1
  Pipe (MA)/RConn1 -- Pipe (MA)1/LConn1 -- A/RConn1

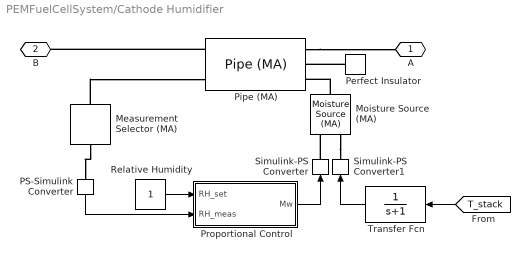
== system PEMFuelCellSystem/Cathode Humidifier ==
  Measurement Selector (MA) : fl_lib/Moist Air/Sensors/Measurement Selector (MA)  moisture_spec=foundation.enum.moisture_spec.relative_humidity  trace_gas_spec=foundation.enum.trace_gas_spec.mole_fraction
      settings: InternalSimscapePortConfiguration="{\"Bottom\":[],\"Left\":[{\"id\":\"F\",\"label\":\"F\",\"type\":\"input\"}],\"Right\":[{\"id\":\"P\",\"label\":\"P\",\"type\":\"output\"},{\"id\":\"T\",\"label\":\"T\",\"type\":\"output\"},{\"id\":\"W\",\"label\":\"W\",\"type\":\"output\"},{\"id\":\"G\",\"label\":\"G\",\"type\":\"output\"},{\"id\":\"D\",\"label\":\"D\",\"type\":\"output\"}],\"Top\":[]}"
  Moisture Source (MA) : fl_lib/Moist Air/Sources/Moisture & Trace Gas Sources/Moisture Source (MA)  source_type=foundation.enum.constant_controlled.controlled  moisture_source_spec=foundation.enum.MoistureSourceSpec.WaterVapor  vapor_from_liquid=false  moisture_mass_flow=0 kg/s  temperature_spec=foundation.enum.temperature_spec.atmospheric  moisture_temperature=293.15 K  Phi_S_specify=off  Phi_S_priority=None  Phi_S=0 kW  Phi_S_nominal_specify=off  Phi_S_nominal_value=1  Phi_S_nominal_unit=kW  mdot_w_S_specify=off  mdot_w_S_priority=None  mdot_w_S=0 kg/s  mdot_w_S_nominal_specify=off  mdot_w_S_nominal_value=1  mdot_w_S_nominal_unit=kg/s  mdot_d_S_specify=off  mdot_d_S_priority=None  mdot_d_S=0 kg/s  mdot_d_S_nominal_specify=off  mdot_d_S_nominal_value=1  mdot_d_S_nominal_unit=kg/s
      settings: InternalSimscapePortConfiguration="{\"Bottom\":[],\"Left\":[{\"id\":\"S\",\"label\":\"S\",\"type\":\"foundation.moist_air.moist_air_source\"}],\"Right\":[{\"id\":\"M\",\"label\":\"M\",\"type\":\"input\"},{\"id\":\"T\",\"label\":\"T\",\"type\":\"input\"}],\"Top\":[]}"
  PS-Simulink Converter : nesl_utility/PS-Simulink Converter  PhysicalDomain=network_engine_domain  SubClassName=ps_output  LeftPortType=input  RightPortType=output  PseudoPeriodic=off  Frequencies=[]  VectorFormat=1-D array  Unit=1  AffineConversion=off
  Perfect Insulator : fl_lib/Thermal/Thermal Elements/Perfect Insulator  T_specify=off  T_priority=None  T=0 K  T_nominal_specify=off  T_nominal_value=1  T_nominal_unit=K
  Pipe (MA) : fl_lib/Moist Air/Elements/Pipe (MA)  length=0.25 m  area=pi*0.05^2/4 m^2  Dh=0.05 m  length_add=0.1 m  roughness=15e-6 m  Re_lam=2000  Re_tur=4000  shape_factor=64  Nu_lam=3.66  wall_condensation=simscape.enum.onoff.off  RH_ws=1  time_constant_cond=1e-3 s  time_constant_evap=1e-3 s  fraction_entrained=1  moisture_trace_gas_source=foundation.enum.moisture_trace_gas_source.controlled  moisture_source_spec=foundation.enum.MoistureSourceSpec.WaterVapor  vapor_from_liquid=false  moisture_mass_flow=0 kg/s  moisture_temperature_spec=foundation.enum.temperature_spec.atmospheric  moisture_temperature=293.15 K  trace_gas_mass_flow=0 kg/s  trace_gas_temperature_spec=foundation.enum.temperature_spec.atmospheric  trace_gas_temperature=293.15 K  p_init=env_p MPa  p_init_priority=foundation.enum.Priority.High  T_init=env_T degC  T_init_priority=foundation.enum.Priority.High  humidity_spec=foundation.enum.HumiditySpec.RelativeHumidity  RH_init=env_RH  RH_init_priority=foundation.enum.Priority.High  x_w_init=0  x_w_init_priority=foundation.enum.Priority.None  y_w_init=0  y_w_init_priority=foundation.enum.Priority.None  HR_init=0  HR_init_priority=foundation.enum.Priority.None  Tw_init=287 K  Tw_init_priority=foundation.enum.Priority.High  trace_gas_spec=foundation.enum.trace_gas_spec.mole_fraction  x_g_init=0  x_g_init_priority=foundation.enum.Priority.None  y_g_init=env_yO2  y_g_init_priority=foundation.enum.Priority.High  r_d_init=0  r_d_init_priority=foundation.enum.Priority.High
      settings: InternalSimscapePortConfiguration="{\"Bottom\":[],\"Left\":[{\"id\":\"A\",\"label\":\"A\",\"type\":\"foundation.moist_air.moist_air\"},{\"id\":\"H\",\"label\":\"H\",\"type\":\"foundation.thermal.thermal\"},{\"id\":\"S\",\"label\":\"S\",\"type\":\"foundation.moist_air.moist_air_source\"}],\"Right\":[{\"id\":\"B\",\"label\":\"B\",\"type\":\"foundation.moist_air.moist_air\"},{\"id\":\"W\",\"label\":\"W\",\"type\":\"output\"},{\"id\":\"F\",\"label\":\"F\",\"type\":\"output\"}],\"Top\":[]}"
  Proportional Control : Subsystem
  Relative Humidity : Constant
  Simulink-PS Converter : nesl_utility/Simulink-PS Converter  PhysicalDomain=network_engine_domain  SubClassName=ps_input  LeftPortType=input  RightPortType=output  PseudoPeriodic=off  Frequencies=[]  NoiseDistribution=none  NoiseParameters=[]  Unit=kg/s  AffineConversion=off  FilteringAndDerivatives=provide  SimscapeFilterOrder=1  InputFilterTimeConstant=0.001  UdotUserProvided=0
  Simulink-PS Converter1 : nesl_utility/Simulink-PS Converter  PhysicalDomain=network_engine_domain  SubClassName=ps_input  LeftPortType=input  RightPortType=output  PseudoPeriodic=off  Frequencies=[]  NoiseDistribution=none  NoiseParameters=[]  Unit=degC  AffineConversion=on  FilteringAndDerivatives=provide  SimscapeFilterOrder=1  InputFilterTimeConstant=0.001  UdotUserProvided=0
  Transfer Fcn : TransferFcn  Denominator=[1 1]
  A : PMIOPort  Side=Right
  B : PMIOPort  Port=2  Side=Left
  wires:
  Transfer Fcn/1 -> Simulink-PS Converter1/1
  [T_stack] -> Transfer Fcn/1
  Proportional Control/1(Mw) -> Simulink-PS Converter/1
  Relative Humidity/1 -> Proportional Control/1(RH_set)
  PS-Simulink Converter/1 -> Proportional Control/2(RH_meas)
  connections:
  Moisture Source (MA)/RConn2 -- Simulink-PS Converter1/RConn1
  Measurement Selector (MA)/LConn1 -- Pipe (MA)/RConn3
  Simulink-PS Converter/RConn1 -- Moisture Source (MA)/RConn1
  Perfect Insulator/LConn1 -- Pipe (MA)/LConn2
  Measurement Selector (MA)/RConn3 -- PS-Simulink Converter/LConn1
  Moisture Source (MA)/LConn1 -- Pipe (MA)/LConn3
  Pipe (MA)/RConn1 -- B/RConn1
  Pipe (MA)/LConn1 -- A/RConn1

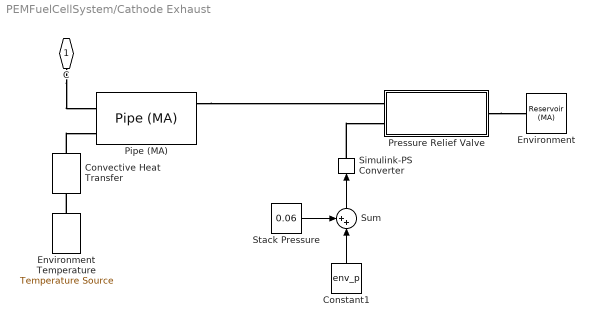
== system PEMFuelCellSystem/Cathode Exhaust ==
  Constant1 : Constant  Value=env_p
  Convective Heat Transfer : fl_lib/Thermal/Thermal Elements/Convective Heat Transfer  thermal_type=foundation.enum.constant_variable.constant  area=pi*cathode_tube_D*1 m^2  heat_tr_coeff=20 W/(m^2 * K)  min_heat_tr_coeff=1e-3 W/(K*m^2)  T_specify=off  T_priority=None  T=0 K  T_nominal_specify=off  T_nominal_value=1  T_nominal_unit=K  Q_specify=off  Q_priority=None  Q=0 W  Q_nominal_specify=off  Q_nominal_value=1  Q_nominal_unit=W
  Environment : fl_lib/Moist Air/Elements/Reservoir (MA)  pressure_input=false  pressure_spec=foundation.enum.pressure_spec.specified  reservoir_pressure=env_p MPa  temperature_input=false  temperature_spec=foundation.enum.temperature_spec.specified  reservoir_temperature=env_T degC  humidity_input=false  humidity_spec=foundation.enum.HumiditySpec.RelativeHumidity  reservoir_RH=env_RH  reservoir_x_w=0.01  reservoir_y_w=0.01  reservoir_HR=0.01  reservoir_Tw=287 K  trace_gas_input=false  trace_gas_spec=foundation.enum.trace_gas_spec.mole_fraction  reservoir_x_g=0.001  reservoir_y_g=env_yO2  water_droplets_input=false  reservoir_r_d=0  RH_ws=1  area_A=pi*cathode_tube_D^2/4 m^2  input_error_spec=foundation.enum.input_range_error.warn
  Environment Temperature : fl_lib/Thermal/Thermal Sources/Temperature Source  temperature=env_T degC
  Pipe (MA) : fl_lib/Moist Air/Elements/Pipe (MA)  length=1 m  area=pi*cathode_tube_D^2/4 m^2  Dh=cathode_tube_D m  length_add=0.1 m  roughness=15e-6 m  Re_lam=2000  Re_tur=4000  shape_factor=64  Nu_lam=3.66  wall_condensation=simscape.enum.onoff.off  RH_ws=1  time_constant_cond=1e-3 s  time_constant_evap=1e-3 s  fraction_entrained=1  moisture_trace_gas_source=foundation.enum.moisture_trace_gas_source.none  moisture_source_spec=foundation.enum.MoistureSourceSpec.WaterVapor  vapor_from_liquid=false  moisture_mass_flow=0 kg/s  moisture_temperature_spec=foundation.enum.temperature_spec.atmospheric  moisture_temperature=293.15 K  trace_gas_mass_flow=0 kg/s  trace_gas_temperature_spec=foundation.enum.temperature_spec.atmospheric  trace_gas_temperature=293.15 K  p_init=env_p MPa  p_init_priority=foundation.enum.Priority.High  T_init=env_T degC  T_init_priority=foundation.enum.Priority.High  humidity_spec=foundation.enum.HumiditySpec.RelativeHumidity  RH_init=env_RH  RH_init_priority=foundation.enum.Priority.High  x_w_init=0  x_w_init_priority=foundation.enum.Priority.None  y_w_init=0  y_w_init_priority=foundation.enum.Priority.None  HR_init=0  HR_init_priority=foundation.enum.Priority.None  Tw_init=287 K  Tw_init_priority=foundation.enum.Priority.High  trace_gas_spec=foundation.enum.trace_gas_spec.mole_fraction  x_g_init=0  x_g_init_priority=foundation.enum.Priority.None  y_g_init=env_yO2  y_g_init_priority=foundation.enum.Priority.High  r_d_init=0  r_d_init_priority=foundation.enum.Priority.High
  Pressure Relief Valve : Subsystem  Tag=PublishSubsystem  mask(Pressure Relief Valve){D=cathode_tube_D, r_min=1e-4, r_max=0.8, p_range=0.005}
      mask prompts: D "Connecting tube diameter (m)"; r_min "Min diameter ratio"; r_max "Max diameter ratio"; p_range "Pressure regulation range (MPa)"
      mask help: This subsystem models a pressure relief valve that maintains a set pressure at port A. The valve is normally closed. When the pressure is above the set pressure, it begins to open.
  Simulink-PS Converter : nesl_utility/Simulink-PS Converter  PhysicalDomain=network_engine_domain  SubClassName=ps_input  LeftPortType=input  RightPortType=output  PseudoPeriodic=off  Frequencies=[]  NoiseDistribution=none  NoiseParameters=[]  Unit=MPa  AffineConversion=off  FilteringAndDerivatives=provide  SimscapeFilterOrder=1  InputFilterTimeConstant=0.001  UdotUserProvided=0
  Stack Pressure : Constant  Value=0.06
  Sum : Sum  Inputs=++|
  C : PMIOPort  Side=Left
  wires:
  Stack Pressure/1 -> Sum/1
  Sum/1 -> Simulink-PS Converter/1
  Constant1/1 -> Sum/2
  connections:
  Pipe (MA)/RConn1 -- Pressure Relief Valve/LConn1
  C/RConn1 -- Pipe (MA)/LConn1
  Convective Heat Transfer/LConn1 -- Pipe (MA)/LConn2
  Environment Temperature/LConn1 -- Convective Heat Transfer/RConn1
  Pressure Relief Valve/RConn1 -- Environment/LConn1
  Simulink-PS Converter/RConn1 -- Pressure Relief Valve/LConn2

== system PEMFuelCellSystem/Cathode Gas Channels ==
  note: connection to share cathode fluid properties only
  Pipe (MA) : fl_lib/Moist Air/Elements/Pipe (MA)  length=sqrt(stack_area) / 2 cm  area=stack_w_channels^2 * stack_num_channels * stack_num_cells cm^2  Dh=stack_w_channels cm  length_add=1 cm  roughness=15e-6 m  Re_lam=2000  Re_tur=4000  shape_factor=64  Nu_lam=3.66  wall_condensation=simscape.enum.onoff.off  RH_ws=1  time_constant_cond=1e-3 s  time_constant_evap=1e-3 s  fraction_entrained=1  moisture_trace_gas_source=foundation.enum.moisture_trace_gas_source.none  moisture_source_spec=foundation.enum.MoistureSourceSpec.WaterVapor  vapor_from_liquid=false  moisture_mass_flow=0 kg/s  moisture_temperature_spec=foundation.enum.temperature_spec.atmospheric  moisture_temperature=293.15 K  trace_gas_mass_flow=0 kg/s  trace_gas_temperature_spec=foundation.enum.temperature_spec.atmospheric  trace_gas_temperature=293.15 K  p_init=env_p MPa  p_init_priority=foundation.enum.Priority.High  T_init=env_T degC  T_init_priority=foundation.enum.Priority.High  humidity_spec=foundation.enum.HumiditySpec.RelativeHumidity  RH_init=env_RH  RH_init_priority=foundation.enum.Priority.High  x_w_init=0  x_w_init_priority=foundation.enum.Priority.None  y_w_init=0  y_w_init_priority=foundation.enum.Priority.None  HR_init=0  HR_init_priority=foundation.enum.Priority.None  Tw_init=287 K  Tw_init_priority=foundation.enum.Priority.High  trace_gas_spec=foundation.enum.trace_gas_spec.mole_fraction  x_g_init=0  x_g_init_priority=foundation.enum.Priority.None  y_g_init=env_yO2  y_g_init_priority=foundation.enum.Priority.High  r_d_init=0  r_d_init_priority=foundation.enum.Priority.High
  Pipe (MA)1 : fl_lib/Moist Air/Elements/Pipe (MA)  length=sqrt(stack_area) / 2 cm  area=stack_w_channels^2 * stack_num_channels * stack_num_cells cm^2  Dh=stack_w_channels cm  length_add=1 cm  roughness=15e-6 m  Re_lam=2000  Re_tur=4000  shape_factor=64  Nu_lam=3.66  wall_condensation=simscape.enum.onoff.off  RH_ws=1  time_constant_cond=1e-3 s  time_constant_evap=1e-3 s  fraction_entrained=1  moisture_trace_gas_source=foundation.enum.moisture_trace_gas_source.controlled  moisture_source_spec=foundation.enum.MoistureSourceSpec.WaterVapor  vapor_from_liquid=false  moisture_mass_flow=0 kg/s  moisture_temperature_spec=foundation.enum.temperature_spec.atmospheric  moisture_temperature=293.15 K  trace_gas_mass_flow=0 kg/s  trace_gas_temperature_spec=foundation.enum.temperature_spec.atmospheric  trace_gas_temperature=293.15 K  p_init=env_p MPa  p_init_priority=foundation.enum.Priority.High  T_init=env_T degC  T_init_priority=foundation.enum.Priority.High  humidity_spec=foundation.enum.HumiditySpec.RelativeHumidity  RH_init=env_RH  RH_init_priority=foundation.enum.Priority.High  x_w_init=0  x_w_init_priority=foundation.enum.Priority.None  y_w_init=0  y_w_init_priority=foundation.enum.Priority.None  HR_init=0  HR_init_priority=foundation.enum.Priority.None  Tw_init=287 K  Tw_init_priority=foundation.enum.Priority.High  trace_gas_spec=foundation.enum.trace_gas_spec.mole_fraction  x_g_init=0  x_g_init_priority=foundation.enum.Priority.None  y_g_init=env_yO2  y_g_init_priority=foundation.enum.Priority.High  r_d_init=0  r_d_init_priority=foundation.enum.Priority.High
      settings: InternalSimscapePortConfiguration="{\"Bottom\":[],\"Left\":[{\"id\":\"A\",\"label\":\"A\",\"type\":\"foundation.moist_air.moist_air\"},{\"id\":\"H\",\"label\":\"H\",\"type\":\"foundation.thermal.thermal\"},{\"id\":\"S\",\"label\":\"S\",\"type\":\"foundation.moist_air.moist_air_source\"}],\"Right\":[{\"id\":\"B\",\"label\":\"B\",\"type\":\"foundation.moist_air.moist_air\"},{\"id\":\"W\",\"label\":\"W\",\"type\":\"output\"},{\"id\":\"F\",\"label\":\"F\",\"type\":\"output\"}],\"Top\":[]}"
  C : PMIOPort  Side=Left
  SC : PMIOPort  Port=2  Side=Left
  FCi : PMIOPort  Port=3  Side=Left
  in : PMIOPort  Port=4  Side=Right
  out : PMIOPort  Port=5  Side=Right
  H : PMIOPort  Port=6  Side=Right
  FCo : PMIOPort  Port=7  Side=Left
  connections:
  Pipe (MA)/LConn1 -- in/RConn1
  Pipe (MA)1/RConn1 -- out/RConn1
  Pipe (MA)/LConn2 -- Pipe (MA)1/LConn2 -- H/RConn1
  Pipe (MA)1/RConn3 -- FCo/RConn1
  Pipe (MA)1/LConn3 -- SC/RConn1
  Pipe (MA)/RConn1 -- C/RConn1 -- Pipe (MA)1/LConn1
  Pipe (MA)/RConn3 -- FCi/RConn1
